simulink model "Car_Parking"  (R2020a)
settings: Solver=VariableStepAuto  StartTime=0.0  StopTime=100  RelTol=1e-3
model workspace: external: MAT-File (data not in the file)
settings Model: EnablePacing=on  OrderedModelArguments=off  Creator=User  LastModifiedBy=User

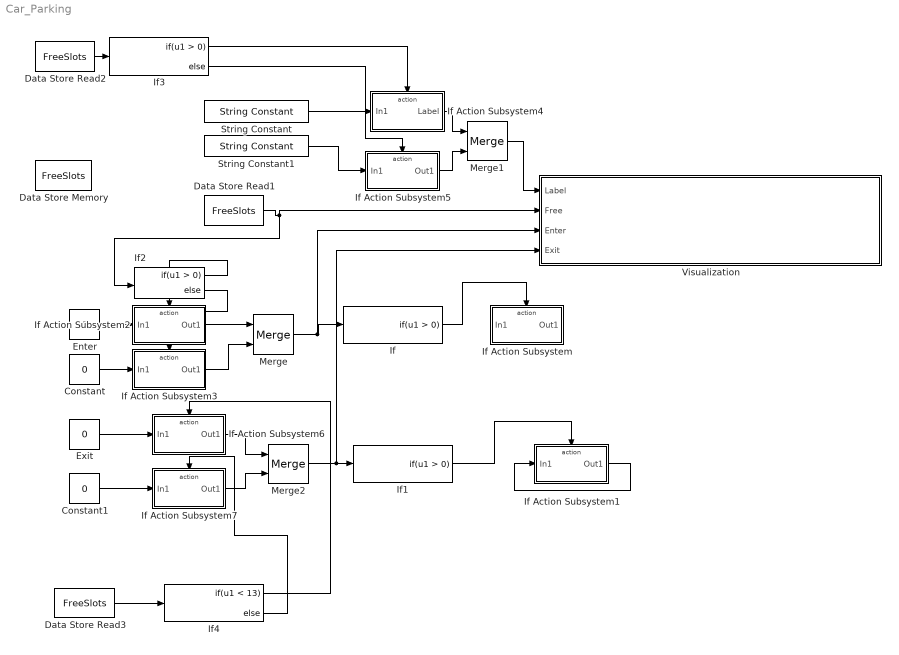
== system Car_Parking ==
  Constant : Constant  Value=0
  Constant1 : Constant  Value=0
  Data Store Memory : DataStoreMemory  DataStoreName=FreeSlots  ReadBeforeWriteMsg=warning  WriteAfterWriteMsg=warning  WriteAfterReadMsg=warning  InitialValue=13  ShowAdditionalParam=off  OutMin=0  OutMax=13  OutDataTypeStr=int8  Dimensions=1
  Data Store Read1 : DataStoreRead  DataStoreName=FreeSlots  SampleTime=1
  Data Store Read2 : DataStoreRead  DataStoreName=FreeSlots  SampleTime=1
  Data Store Read3 : DataStoreRead  DataStoreName=FreeSlots  SampleTime=1
  Enter : Constant  Value=0
  Exit : Constant  Value=0
  If : If  ShowElse=off
  If Action Subsystem : Subsystem  TreatAsAtomicUnit=on
  If Action Subsystem1 : Subsystem  TreatAsAtomicUnit=on
  If Action Subsystem2 : Subsystem  TreatAsAtomicUnit=on
  If Action Subsystem3 : Subsystem  TreatAsAtomicUnit=on
  If Action Subsystem4 : Subsystem  TreatAsAtomicUnit=on
  If Action Subsystem5 : Subsystem  TreatAsAtomicUnit=on
  If Action Subsystem6 : Subsystem  TreatAsAtomicUnit=on
  If Action Subsystem7 : Subsystem  TreatAsAtomicUnit=on
  If1 : If  ShowElse=off
  If2 : If
  If3 : If
  If4 : If  IfExpression=u1 < 13
  Merge : Merge
  Merge1 : Merge
  Merge2 : Merge
  String Constant : StringConstant  String="\"Welcome!!!\""
  String Constant1 : StringConstant  String="\"Please Come Later!!!\""
  Visualization : Subsystem
      mask Display: disp("Double click me to see the visualization")
  wires:
  Data Store Read1/1 -> If2/1, Visualization/2(Free)
  If/1 -> If Action Subsystem/Action
  Enter/1 -> If Action Subsystem2/1(In1)
  If1/1 -> If Action Subsystem1/Action
  If2/1 -> If Action Subsystem2/Action
  Constant/1 -> If Action Subsystem3/1(In1)
  If2/2 -> If Action Subsystem3/Action
  If Action Subsystem2/1(Out1) -> Merge/1
  If Action Subsystem3/1(Out1) -> Merge/2
  Merge/1 -> Visualization/3(Enter), If/1
  String Constant/1 -> If Action Subsystem4/1(In1)
  If3/1 -> If Action Subsystem4/Action
  String Constant1/1 -> If Action Subsystem5/1(In1)
  If Action Subsystem4/1(Label) -> Merge1/1
  If Action Subsystem5/1(Out1) -> Merge1/2
  Merge1/1 -> Visualization/1(Label)
  If3/2 -> If Action Subsystem5/Action
  If Action Subsystem1/1(Out1) -> If Action Subsystem1/1(In1)
  Data Store Read2/1 -> If3/1
  Data Store Read3/1 -> If4/1
  Exit/1 -> If Action Subsystem6/1(In1)
  If4/1 -> If Action Subsystem6/Action
  If Action Subsystem6/1(Out1) -> Merge2/1
  Merge2/1 -> Visualization/4(Exit), If1/1
  If Action Subsystem7/1(Out1) -> Merge2/2
  If4/2 -> If Action Subsystem7/Action
  Constant1/1 -> If Action Subsystem7/1(In1)

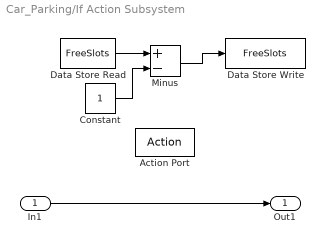
== system Car_Parking/If Action Subsystem ==
  In1 : Inport
  Action Port : ActionPort  ActionPortLabel=if(u1 > 0)
  Constant : Constant  OutDataTypeStr=int8
  Data Store Read : DataStoreRead  DataStoreName=FreeSlots
  Data Store Write : DataStoreWrite  DataStoreName=FreeSlots  DataStoreElements=FreeSlots
  Minus : Sum  Inputs=+-
  Out1 : Outport
  wires:
  Minus/1 -> Data Store Write/1
  Data Store Read/1 -> Minus/1
  Constant/1 -> Minus/2
  In1/1 -> Out1/1

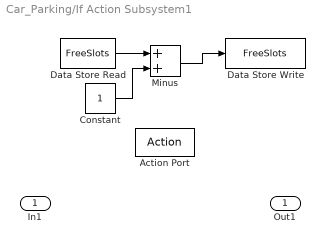
== system Car_Parking/If Action Subsystem1 ==
  In1 : Inport
  Action Port : ActionPort  ActionPortLabel=if(u1 > 0)
  Constant : Constant  OutDataTypeStr=int8
  Data Store Read : DataStoreRead  DataStoreName=FreeSlots
  Data Store Write : DataStoreWrite  DataStoreName=FreeSlots  DataStoreElements=FreeSlots
  Minus : Sum
  Out1 : Outport
  wires:
  Minus/1 -> Data Store Write/1
  Data Store Read/1 -> Minus/1
  Constant/1 -> Minus/2

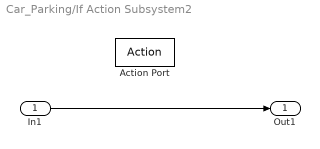
== system Car_Parking/If Action Subsystem2 ==
  In1 : Inport
  Action Port : ActionPort  ActionPortLabel=if(u1 > 0)
  Out1 : Outport
  wires:
  In1/1 -> Out1/1

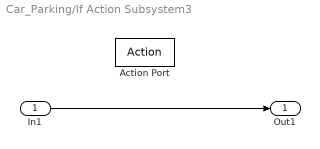
== system Car_Parking/If Action Subsystem3 ==
  In1 : Inport
  Action Port : ActionPort  ActionPortLabel=else
  Out1 : Outport
  wires:
  In1/1 -> Out1/1

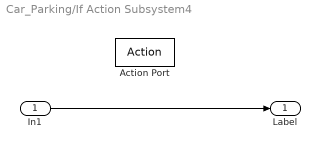
== system Car_Parking/If Action Subsystem4 ==
  In1 : Inport
  Action Port : ActionPort  ActionPortLabel=if(u1 > 0)
  Label : Outport
  wires:
  In1/1 -> Label/1

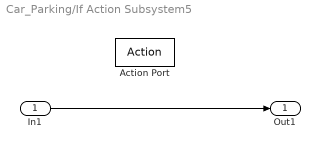
== system Car_Parking/If Action Subsystem5 ==
  In1 : Inport
  Action Port : ActionPort  ActionPortLabel=else
  Out1 : Outport
  wires:
  In1/1 -> Out1/1

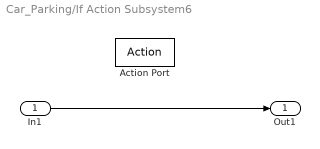
== system Car_Parking/If Action Subsystem6 ==
  In1 : Inport
  Action Port : ActionPort  ActionPortLabel=if(u1 < 13)
  Out1 : Outport
  wires:
  In1/1 -> Out1/1

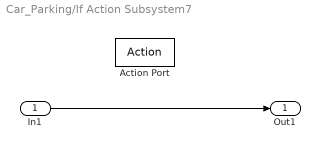
== system Car_Parking/If Action Subsystem7 ==
  In1 : Inport
  Action Port : ActionPort  ActionPortLabel=else
  Out1 : Outport
  wires:
  In1/1 -> Out1/1

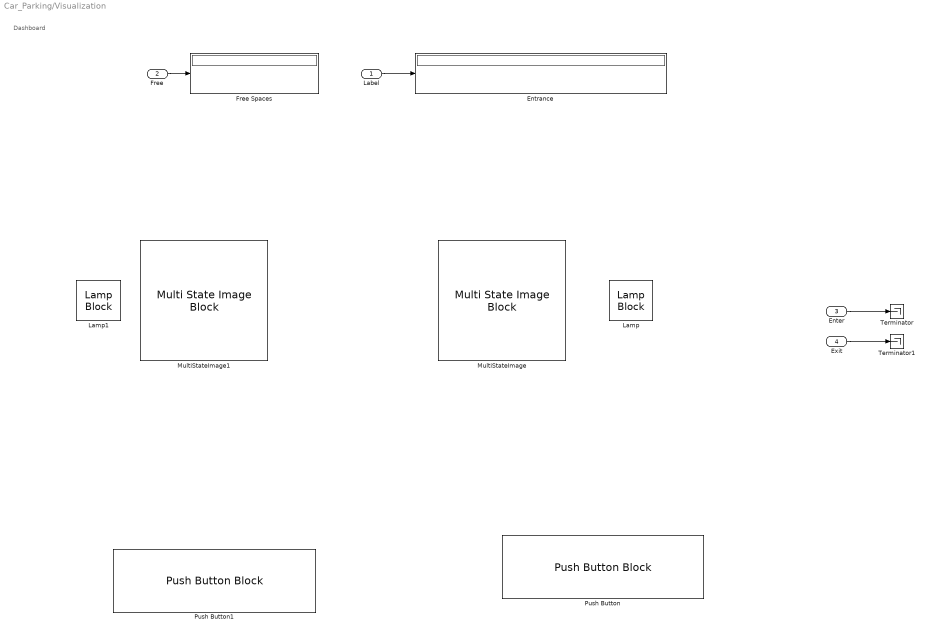
== system Car_Parking/Visualization ==
  note: Dashboard
  Label : Inport
  Free : Inport  Port=2
  Enter : Inport  Port=3
  Exit : Inport  Port=4
  Entrance : Display
  Free Spaces : Display
  Lamp : LampBlock  LabelPosition=Hide
  Lamp1 : LampBlock  LabelPosition=Hide
  MultiStateImage : MultiStateImageBlock  LabelPosition=Hide
  MultiStateImage1 : MultiStateImageBlock  LabelPosition=Hide
  Push Button : PushButtonBlock  ButtonText=Push to Enter
  Push Button1 : PushButtonBlock  ButtonText=Push to Exit
  Terminator : Terminator
  Terminator1 : Terminator
  wires:
  Label/1 -> Entrance/1
  Enter/1 -> Terminator/1
  Free/1 -> Free Spaces/1
  Exit/1 -> Terminator1/1
